simulink subsystem "randomupc"  (R2020b)
settings: Solver=VariableStepAuto  StartTime=0.0  StopTime=10.0  RelTol=1e-3
settings Model: Creator=billy  LastModifiedBy=billy

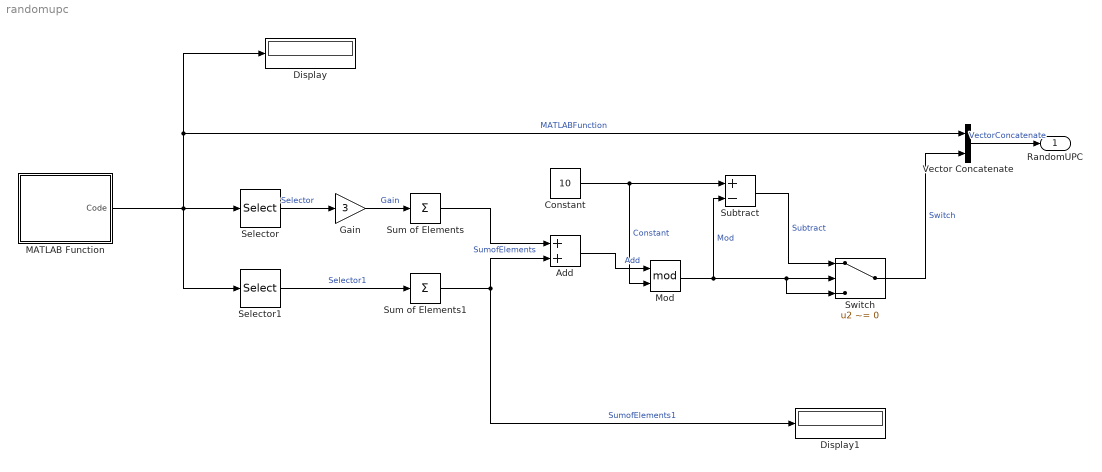
== system randomupc ==
  Add : Sum
  Constant : Constant  Value=10
  Display : Display
  Display1 : Display
  Gain : Gain  Gain=3
  MATLAB Function : MATLAB Function  TreatAsAtomicUnit=on
  Mod : Math  Operator=mod  SaturateOnIntegerOverflow=on
  Selector : Selector  InputPortWidth=11  IndexOptions=Index vector (dialog)  Indices=[1 3 5 7 9 11]  OutputSizes=1
  Selector1 : Selector  IndexMode=Zero-based  InputPortWidth=11  IndexOptions=Index vector (dialog)  Indices=[2 4 6 8 10]  OutputSizes=1
  Subtract : Sum  Inputs=+-
  Sum of Elements : Sum  Inputs=+
  Sum of Elements1 : Sum  Inputs=+
  Switch : Switch  Criteria=u2 ~= 0
  Vector Concatenate : Concatenate
  RandomUPC : Outport
  wires:
  Selector1/1 -> Sum of Elements1/1  "Selector1"
  MATLAB Function/1(Code) -> Vector Concatenate/1, Display/1, Selector1/1, Selector/1  "MATLABFunction"
  Sum of Elements/1 -> Add/1  "SumofElements"
  Gain/1 -> Sum of Elements/1  "Gain"
  Sum of Elements1/1 -> Display1/1, Add/2  "SumofElements1"
  Constant/1 -> Mod/2, Subtract/1  "Constant"
  Add/1 -> Mod/1  "Add"
  Selector/1 -> Gain/1  "Selector"
  Mod/1 -> Subtract/2, Switch/3, Switch/2  "Mod"
  Subtract/1 -> Switch/1  "Subtract"
  Vector Concatenate/1 -> RandomUPC/1  "VectorConcatenate"
  Switch/1 -> Vector Concatenate/2  "Switch"

== matlab function randomupc/MATLAB Function ==
  data: Code output
function Code = IncompleteCode
    Code = randi([0 9], 1, 11)
end
